simulink model "buck_ssm"  (R2021a)
settings: Solver=VariableStepAuto  StartTime=0.0  StopTime=10.0  RelTol=1e-3
values from neighbouring files (symbols this model uses):
  C = ( irip * Ts ) / (8 * vrip)    (= 5.20833333333e-06)    [lsm.m]
  D = (V)/(Vg-(Iout*Rg))    (= 0.447204968944)    [lsm.m]
  Iout = Pout/V    (= 8.33333333333)    [lsm.m]
  L = ((Vg - V) / (2*irip)) * D * Ts    (= 8.58633540373e-05)    [lsm.m]
  Rg = 140e-3    (= 0.14)    [lsm.m]
  Rl = V/Iout    (= 1.44)    [lsm.m]
  Vg = 28    [lsm.m]
libraries: spsSeriesRLCBranchLib x4, spsControlledCurrentSourceLib x3, spsGroundLib x3, spsControlledVoltageSourceLib x2, spsCurrentMeasurementLib x1, spsDCVoltageSourceLib x1, spsVoltageMeasurementLib x1, spspowerguiLib x1
settings Model: Creator=yoshi  LastModifiedBy=yoshi

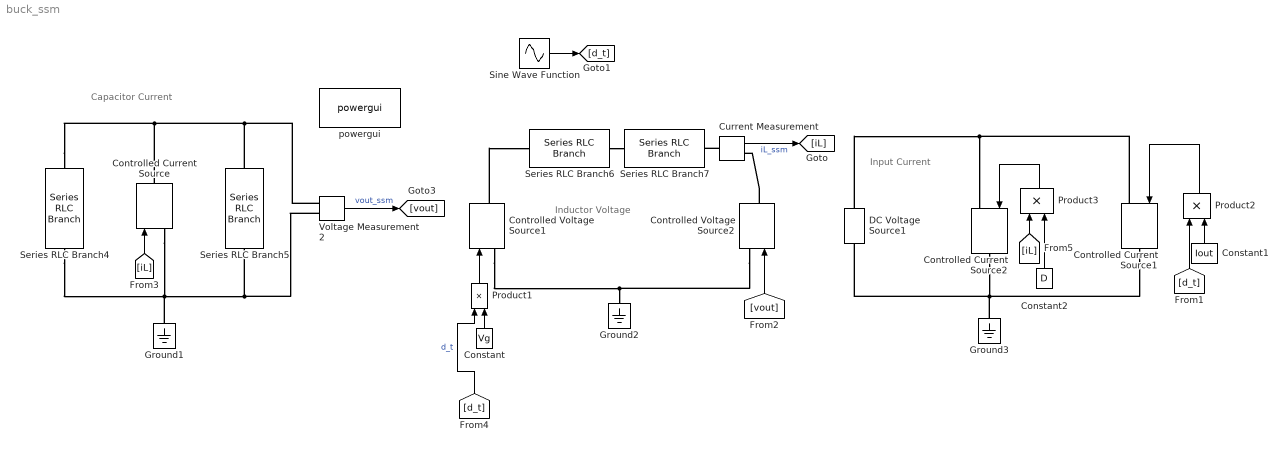
== system buck_ssm ==
  note: Capacitor Current
  note: Input Current
  note: Inductor Voltage
  Constant : Constant  Value=Vg
  Constant1 : Constant  Value=Iout
  Constant2 : Constant  Value=D
  Controlled Current Source : spsControlledCurrentSourceLib/Controlled Current Source  Initialize=on  Source_Type=AC  Amplitude=0  Phase=0  Frequency=0  Measurements=None
  Controlled Current Source1 : spsControlledCurrentSourceLib/Controlled Current Source  Initialize=on  Source_Type=AC  Amplitude=0  Phase=0  Frequency=0  Measurements=None
  Controlled Current Source2 : spsControlledCurrentSourceLib/Controlled Current Source  Initialize=on  Source_Type=AC  Amplitude=0  Phase=0  Frequency=0  Measurements=None
  Controlled Voltage Source1 : spsControlledVoltageSourceLib/Controlled Voltage Source  Initialize=on  Source_Type=AC  Amplitude=0  Phase=0  Frequency=0  Measurements=None
  Controlled Voltage Source2 : spsControlledVoltageSourceLib/Controlled Voltage Source  Initialize=on  Source_Type=AC  Amplitude=0  Phase=0  Frequency=0  Measurements=None
  Current Measurement : spsCurrentMeasurementLib/Current Measurement  PhasorSimulation=off  OutputType=Complex  PSBequivalent=0
  DC Voltage Source1 : spsDCVoltageSourceLib/DC Voltage Source  Amplitude=Vg  Measurements=None
  Ground1 : spsGroundLib/Ground  LConnTagsString=a
  Ground2 : spsGroundLib/Ground  LConnTagsString=a
  Ground3 : spsGroundLib/Ground  LConnTagsString=a
  Product1 : Product
  Product2 : Product
  Product3 : Product
  Series RLC Branch4 : spsSeriesRLCBranchLib/Series RLC Branch  LConnTagsString=__new0  RConnTagsString=__new0  BranchType=C  Resistance=1  Inductance=1e-3  SetiL0=off  InitialCurrent=0  Capacitance=C  Setx0=off  InitialVoltage=0  Measurements=None
  Series RLC Branch5 : spsSeriesRLCBranchLib/Series RLC Branch  LConnTagsString=__new0  RConnTagsString=__new0  BranchType=R  Resistance=Rl  Inductance=1e-3  SetiL0=off  InitialCurrent=0  Capacitance=1e-6  Setx0=off  InitialVoltage=0  Measurements=None
  Series RLC Branch6 : spsSeriesRLCBranchLib/Series RLC Branch  LConnTagsString=__new0  RConnTagsString=__new0  BranchType=R  Resistance=Rg  Inductance=1e-3  SetiL0=off  InitialCurrent=0  Capacitance=1e-6  Setx0=off  InitialVoltage=0  Measurements=None
  Series RLC Branch7 : spsSeriesRLCBranchLib/Series RLC Branch  LConnTagsString=__new0  RConnTagsString=__new0  BranchType=L  Resistance=1  Inductance=L  SetiL0=off  InitialCurrent=0  Capacitance=1e-6  Setx0=off  InitialVoltage=0  Measurements=None
  Sine Wave Function : Sin  Amplitude=0.1  Frequency=2*pi*60  SampleTime=0
  Voltage Measurement2 : spsVoltageMeasurementLib/Voltage Measurement  PhasorSimulation=off  OutputType=Complex  PSBequivalent=0
  powergui : spspowerguiLib/powergui  Priority=1  SimulationMode=Continuous  SampleTime=50e-6  frequency=60  Iterations=50  frequencyindice=0  Pbase=100e6  ErrMax=1e-4  UnitsV=kV  UnitsW=MW  buscounter=0  FunctionMessages=off  echomessages=off  EnableUseOfTLC=off  CurrentSourceSwitches=off  DisableSnubberDevices=off  DisableRonSwitches=off  DisableVfSwitches=off  DisplayEquations=off  AutomaticDiscreteSolvers=off  SolverType=Tustin/Backward Euler (TBE)  Interpol=off  ExternalGateDelay=off  methode=off  Ts=100  x0status=blocks  SPID=on  SwTol=0  HookPort=off  NonlinearTolerance=1e-4  nMaxIteration=100  ContinueOnMaxIteration=off  RestoreLinks=warning  ResistiveCurrentMeasurement=off  Frange=[0:2:500]  Ylog=off  Xlog=on  ShowGrid=off  save=off  variable=ZData  structure=0  ZoomFFT=off  StartTime=0.0  cycles=1  DisplayStyle=1  fundamental=60  FreqAxis=off  MaxFrequency=1000  frequencyindicesteady=1  RmsSteady=1  display=off
  wires:
  Voltage Measurement2/1 -> [vout]  "vout_ssm"
  [vout] -> Controlled Voltage Source2/1
  Current Measurement/1 -> [iL]  "iL_ssm"
  [iL] -> Controlled Current Source/1
  Product1/1 -> Controlled Voltage Source1/1
  Constant/1 -> Product1/2
  Sine Wave Function/1 -> [d_t]
  [d_t] -> Product1/1  "d_t"
  Constant1/1 -> Product2/2
  [d_t] -> Product2/1
  Product2/1 -> Controlled Current Source1/1
  [iL] -> Product3/1
  Constant2/1 -> Product3/2
  Product3/1 -> Controlled Current Source2/1
  connections:
  Series RLC Branch5/RConn1 -- Voltage Measurement2/LConn2 -- Series RLC Branch4/RConn1 -- Ground1/LConn1 -- Controlled Current Source/LConn1
  Series RLC Branch4/LConn1 -- Controlled Current Source/RConn1 -- Series RLC Branch5/LConn1 -- Voltage Measurement2/LConn1
  Controlled Current Source1/RConn1 -- Ground3/LConn1 -- Controlled Current Source2/RConn1 -- DC Voltage Source1/LConn1
  Series RLC Branch6/RConn1 -- Series RLC Branch7/LConn1
  Controlled Voltage Source1/RConn1 -- Series RLC Branch6/LConn1
  Controlled Voltage Source2/LConn1 -- Controlled Voltage Source1/LConn1 -- Ground2/LConn1
  Current Measurement/LConn1 -- Series RLC Branch7/RConn1
  Controlled Voltage Source2/RConn1 -- Current Measurement/RConn1
  Controlled Current Source1/LConn1 -- DC Voltage Source1/RConn1 -- Controlled Current Source2/LConn1
